simulink library "lib_FDM"  (R2019b)
settings: Solver=VariableStepAuto  StartTime=0.0  StopTime=10.0  RelTol=1e-3
values from neighbouring files (symbols this model uses):
  d = config.d_m    [computeTF.m]
undefined symbols (not defined in the file or in its folder): c_b_WGS, c_flat, c_grav, c_rot, c_rsma, Cd0, Cdcl, Cdcl2, Cl0, Cla, Cld, Cma, Cmd, Cmq, Cnb, Cnd, Cnr, Cra, Crd, Crp, Cy0, Cyb, Cyd, dmdt, Earth, HIL_Data, InitThrust, launchPos, me, mf, mp, Sref, tb, TF, theta0, WGS84
libraries: simulink_extras x14, $bdroot x7, simulink x5, lib_Fin_Deflections x3, aerolibasang x2, sharedtransform x1, aerolibtransform2 x1, aerolibbdyn x1, aerolibatmos2 x1, aerolibutil x1, aerolib6dof2 x1
(part 7 of 8)

== system lib_FDM/FDM/FDM_Sophisticated/stream_flow/calc_stream_flow/velocity_vector_transformation/cross_product ==
  note: Inputs [size]:
      |
      | r1 [3x1]
      | r2 [3x1]
  note: Outputs [size]:
      |
      | r1 x r2  [3x1]
  r1 : Inport
  r2 : Inport  Port=2
  Demux2 : Demux  Outputs=[1;1;1]
  Demux3 : Demux  Outputs=[1;1;1]
  Product{2..7} (6 alike) : Product  SaturateOnIntegerOverflow=on  RndMeth=Zero  InputSameDT=on  OutDataTypeStr=Inherit: Same as first input
  Sum : Sum  Inputs=+-  SaturateOnIntegerOverflow=on  InputSameDT=on  OutDataTypeStr=Inherit: Same as first input
  Sum1 : Sum  Inputs=+-  SaturateOnIntegerOverflow=on  InputSameDT=on  OutDataTypeStr=Inherit: Same as first input
  Sum2 : Sum  Inputs=+-  SaturateOnIntegerOverflow=on  InputSameDT=on  OutDataTypeStr=Inherit: Same as first input
  Vector Concatenate : Concatenate  NumInputs=3  Mode=Multidimensional array
  r1_x_r2 : Outport  PortDimensions=[3,1]  VectorParamsAs1DForOutWhenUnconnected=off
  wires:
  Vector Concatenate/1 -> r1_x_r2/1
  r2/1 -> Demux3/1
  r1/1 -> Demux2/1
  Sum2/1 -> Vector Concatenate/3
  Sum1/1 -> Vector Concatenate/2
  Sum/1 -> Vector Concatenate/1
  Product7/1 -> Sum2/2
  Product6/1 -> Sum2/1
  Product5/1 -> Sum1/2
  Product4/1 -> Sum1/1
  Product3/1 -> Sum/2
  Product2/1 -> Sum/1
  Demux2/1 -> Product5/1, Product6/1
  Demux3/1 -> Product4/2, Product7/2
  Demux2/3 -> Product4/1, Product3/1
  Demux3/2 -> Product3/2, Product6/2
  Demux3/3 -> Product2/2, Product5/2
  Demux2/2 -> Product7/1, Product2/1

== system lib_FDM/FDM/FDM_Sophisticated/tmp/weather/atm_dynamic/trafo_around_z_axis ==
  vec1 : Inport
  gamma : Inport  Port=2
  1_rot_mat : Subsystem  mask(Rotation um 1, 2 oder 3 Achsen){rot_1=Rotation um z-Achse}
      mask prompts: rot_1 "1. Rotation"
      mask help:
      | Dieser Block liefert die Rotationsmatrix T12 für den Fall zurück, dass sich das Ziel-Koordinatensystem (1) durch Drehungen um 1, 2 oder 3 Achsen gegenüber dem Ausgangskoordinatensystem (2) beschreiben lässt (passive Drehung).
      |
      | Die Anzahl der Rotation sowie die Reihenfolge ist frei einstellbar.
      |
      | Die Rotationswinkel haben die Einheit [rad].
      mask TypeOptions rot_1: Rotation um x-Achse | Rotation um y-Achse | Rotation um z-Achse
  Product : Product  Multiplication=Matrix(*)
  Reshape : Reshape  OutputDimensionality=Column vector (2-D)
  vec2 : Outport  VectorParamsAs1DForOutWhenUnconnected=off
  wires:
  Reshape/1 -> Product/2  "vec1"
  vec1/1 -> Reshape/1  "vec1"
  1_rot_mat/1(T12) -> Product/1  "T12"
  gamma/1 -> 1_rot_mat/1(wi1)  "gamma"
  Product/1 -> vec2/1  "vec2"

== system lib_FDM/FDM/FDM_Sophisticated/weight_and_balance/moi/moi_coordinate_transformation/3_rot_mat ==
  wi1 : Inport
  wi2 : Inport  Port=2
  wi3 : Inport  Port=3
  1. Rotation x-Achse : Subsystem
  1. Rotation y-Achse : Subsystem
  1. Rotation z-Achse : Subsystem
  2. Rotation x-Achse : Subsystem
  2. Rotation y-Achse : Subsystem
  2. Rotation z-Achse : Subsystem
  3. Rotation : Product  Inputs=***  Multiplication=Matrix(*)
  3. Rotation x-Achse : Subsystem
  3. Rotation y-Achse : Subsystem
  3. Rotation z-Achse : Subsystem
  Constant : Constant  Value=rot_1
  Constant1 : Constant  Value=rot_2
  Constant2 : Constant  Value=rot_3
  Multiport Switch : MultiPortSwitch
  Multiport Switch1 : MultiPortSwitch
  Multiport Switch2 : MultiPortSwitch
  T12 : Outport  VectorParamsAs1DForOutWhenUnconnected=off
  wires:
  3. Rotation x-Achse/1(3Rot_Matrix_x) -> Multiport Switch2/2
  3. Rotation y-Achse/1(3Rot_Matrix_y) -> Multiport Switch2/3
  2. Rotation z-Achse/1(2Rot_Matrix_z) -> Multiport Switch1/4
  2. Rotation y-Achse/1(2Rot_Matrix_y) -> Multiport Switch1/3
  2. Rotation x-Achse/1(2Rot_Matrix_x) -> Multiport Switch1/2
  3. Rotation/1 -> T12/1  "T12"
  Constant2/1 -> Multiport Switch2/1
  1. Rotation z-Achse/1(1Rot_Matrix_z) -> Multiport Switch/4
  1. Rotation y-Achse/1(1Rot_Matrix_y) -> Multiport Switch/3
  Constant1/1 -> Multiport Switch1/1
  1. Rotation x-Achse/1(1Rot_Matrix_x) -> Multiport Switch/2
  Constant/1 -> Multiport Switch/1
  3. Rotation z-Achse/1(3Rot_Matrix_z) -> Multiport Switch2/4
  wi2/1 -> 2. Rotation x-Achse/1(alpha2), 2. Rotation y-Achse/1(alpha2), 2. Rotation z-Achse/1(alpha2)
  wi1/1 -> 1. Rotation x-Achse/1(alpha1), 1. Rotation y-Achse/1(alpha1), 1. Rotation z-Achse/1(alpha1)
  wi3/1 -> 3. Rotation y-Achse/1(alpha3), 3. Rotation z-Achse/1(alpha3), 3. Rotation x-Achse/1(alpha3)
  Multiport Switch/1 -> 3. Rotation/3
  Multiport Switch1/1 -> 3. Rotation/2
  Multiport Switch2/1 -> 3. Rotation/1

== system lib_FDM/FDM/FDM_Sophisticated/weight_and_balance/moi/steiners_theorem_missile/create_deviation_matrix ==
  pBXB : Inport
  Add : Sum
  Add4 : Sum
  Add5 : Sum
  Demux : Demux  Outputs=3
  Gain : Gain  Gain=-1
  Gain1 : Gain  Gain=-1
  Gain3 : Gain  Gain=-1
  Product{1..6} (6 alike) : Product
  Vector Concatenate1 : Concatenate  NumInputs=3  Mode=Multidimensional array  ConcatenateDimension=2
  Vector Concatenate6 : Concatenate  NumInputs=3
  Vector Concatenate7 : Concatenate  NumInputs=3
  Vector Concatenate8 : Concatenate  NumInputs=3
  T_deviation : Outport  VectorParamsAs1DForOutWhenUnconnected=off
  wires:
  pBXB/1 -> Demux/1
  Vector Concatenate8/1 -> Vector Concatenate1/3
  Product3/1 -> Gain/1
  Product4/1 -> Gain1/1
  Gain1/1 -> Vector Concatenate6/3, Vector Concatenate8/1
  Product2/1 -> Add/2, Add4/1
  Product5/1 -> Add5/2, Add4/2
  Product1/1 -> Add/1, Add5/1
  Add/1 -> Vector Concatenate6/1
  Product6/1 -> Gain3/1
  Add5/1 -> Vector Concatenate7/2
  Demux/2 -> Product6/1, Product1/1, Product1/2, Product3/2  "b"
  Vector Concatenate1/1 -> T_deviation/1
  Gain3/1 -> Vector Concatenate7/3, Vector Concatenate8/2
  Gain/1 -> Vector Concatenate6/2, Vector Concatenate7/1
  Demux/3 -> Product2/2, Product2/1, Product4/2, Product6/2  "c"
  Demux/1 -> Product5/1, Product5/2, Product4/1, Product3/1  "a"
  Vector Concatenate7/1 -> Vector Concatenate1/2
  Vector Concatenate6/1 -> Vector Concatenate1/1
  Add4/1 -> Vector Concatenate8/3

== system lib_FDM/FDM/FDM_Sophisticated/weight_and_balance/moi/steiners_theorem_motor/create_deviation_matrix1 ==
  pBXB : Inport
  Add : Sum
  Add4 : Sum
  Add5 : Sum
  Demux : Demux  Outputs=3
  Gain : Gain  Gain=-1
  Gain1 : Gain  Gain=-1
  Gain3 : Gain  Gain=-1
  Product{1..6} (6 alike) : Product
  Vector Concatenate1 : Concatenate  NumInputs=3  Mode=Multidimensional array  ConcatenateDimension=2
  Vector Concatenate6 : Concatenate  NumInputs=3
  Vector Concatenate7 : Concatenate  NumInputs=3
  Vector Concatenate8 : Concatenate  NumInputs=3
  T_deviation : Outport  VectorParamsAs1DForOutWhenUnconnected=off
  wires:
  Add4/1 -> Vector Concatenate8/3
  Vector Concatenate6/1 -> Vector Concatenate1/1
  Vector Concatenate7/1 -> Vector Concatenate1/2
  Demux/1 -> Product3/1, Product4/1, Product5/2, Product5/1  "a"
  Demux/3 -> Product6/2, Product4/2, Product2/1, Product2/2  "c"
  Gain/1 -> Vector Concatenate7/1, Vector Concatenate6/2
  Gain3/1 -> Vector Concatenate8/2, Vector Concatenate7/3
  Vector Concatenate1/1 -> T_deviation/1
  Demux/2 -> Product3/2, Product1/2, Product1/1, Product6/1  "b"
  Add5/1 -> Vector Concatenate7/2
  Product6/1 -> Gain3/1
  Add/1 -> Vector Concatenate6/1
  Product1/1 -> Add5/1, Add/1
  Product5/1 -> Add4/2, Add5/2
  Product2/1 -> Add4/1, Add/2
  Gain1/1 -> Vector Concatenate8/1, Vector Concatenate6/3
  Product4/1 -> Gain1/1
  Product3/1 -> Gain/1
  Vector Concatenate8/1 -> Vector Concatenate1/3
  pBXB/1 -> Demux/1

== system lib_FDM/FDM/FDM_Student/Aerodynamics/-/Calc Thrust/If Action Subsystem ==
  Action Port : ActionPort
  Constant1 : Constant
  Gain : Gain  Gain=[InitThrust, 0, 0]
  Thrust : Outport  VectorParamsAs1DForOutWhenUnconnected=off
  wires:
  Gain/1 -> Thrust/1
  Constant1/1 -> Gain/1

== system lib_FDM/FDM/FDM_Student/Aerodynamics/-/Calc Thrust/If Action Subsystem1 ==
  Action Port : ActionPort
  Constant1 : Constant
  Gain1 : Gain  Gain=[InitThrust*0, 0, 0]
  Thrust1 : Outport  VectorParamsAs1DForOutWhenUnconnected=off
  wires:
  Constant1/1 -> Gain1/1
  Gain1/1 -> Thrust1/1

== system lib_FDM/FDM/FDM_Student/Aerodynamics/Moment Calc/Calc CL Wind/If Action Subsystem ==
  w_Wind : Inport
  delta R : Inport  Port=2
  AOA : Inport  Port=3
  Vb : Inport  Port=4
  Action Port : ActionPort
  C_L_alpha : Gain  Gain=Cra
  C_L_delta : Gain  Gain=Crd
  C_L_p : Gain  Gain=Crp*0.5*d
  Divide : Product  Inputs=*/
  Selector2 : Selector  InputPortWidth=3  IndexOptions=Index vector (dialog)  Indices=1  OutputSizes=1
  Sum1 : Sum  Inputs=|+++
  To Workspace : ToWorkspace  VariableName=Rolling_moment_wind  SaveFormat=Structure  SampleTime=-1
  CL : Outport  VectorParamsAs1DForOutWhenUnconnected=off
  wires:
  C_L_p/1 -> Divide/1
  Divide/1 -> Sum1/1
  C_L_delta/1 -> Sum1/2
  C_L_alpha/1 -> Sum1/3
  w_Wind/1 -> Selector2/1
  delta R/1 -> C_L_delta/1
  AOA/1 -> C_L_alpha/1
  Vb/1 -> Divide/2
  Selector2/1 -> To Workspace/1, C_L_p/1
  Sum1/1 -> CL/1

== system lib_FDM/FDM/FDM_Student/Aerodynamics/Moment Calc/Calc CL Wind/If Action Subsystem1 ==
  Action Port : ActionPort
  Constant : Constant  Value=0  VectorParams1D=off
  CL : Outport  VectorParamsAs1DForOutWhenUnconnected=off
  wires:
  Constant/1 -> CL/1

== system lib_FDM/FDM/FDM_Student/Aerodynamics/Moment Calc/Calc CM Wind/If Action Subsystem2 ==
  alpha : Inport
  delta p : Inport  Port=2
  w_Wind : Inport  Port=3
  Vb : Inport  Port=4
  Action Port : ActionPort
  C_M_alpha : Gain  Gain=Cma
  C_M_delta : Gain  Gain=Cmd
  C_M_q : Gain  Gain=Cmq*0.5*d
  Divide : Product  Inputs=*/
  Selector1 : Selector  InputPortWidth=3  IndexOptions=Index vector (dialog)  Indices=2  OutputSizes=1
  Sum2 : Sum  Inputs=|+++
  CM : Outport  VectorParamsAs1DForOutWhenUnconnected=off
  wires:
  Sum2/1 -> CM/1
  delta p/1 -> C_M_delta/1
  alpha/1 -> C_M_alpha/1
  C_M_alpha/1 -> Sum2/1
  C_M_q/1 -> Divide/1
  C_M_delta/1 -> Sum2/2
  w_Wind/1 -> Selector1/1
  Selector1/1 -> C_M_q/1
  Divide/1 -> Sum2/3
  Vb/1 -> Divide/2

== system lib_FDM/FDM/FDM_Student/Aerodynamics/Moment Calc/Calc CM Wind/If Action Subsystem3 ==
  Action Port : ActionPort
  Constant : Constant  Value=0  VectorParams1D=off
  CM : Outport  VectorParamsAs1DForOutWhenUnconnected=off
  wires:
  Constant/1 -> CM/1

== system lib_FDM/FDM/FDM_Student/Aerodynamics/Moment Calc/Calc CN Wind/If Action Subsystem2 ==
  beta : Inport
  delta Y : Inport  Port=2
  w_Wind : Inport  Port=3
  Vb : Inport  Port=4
  Action Port : ActionPort
  C_N_beta : Gain  Gain=Cnb
  C_N_delta : Gain  Gain=Cnd
  C_N_r : Gain  Gain=Cnr*0.5*d
  Divide1 : Product  Inputs=*/
  Selector1 : Selector  InputPortWidth=3  IndexOptions=Index vector (dialog)  Indices=3  OutputSizes=1
  Sum : Sum  Inputs=|+++
  CN : Outport  VectorParamsAs1DForOutWhenUnconnected=off
  wires:
  w_Wind/1 -> Selector1/1
  delta Y/1 -> C_N_delta/1
  beta/1 -> C_N_beta/1
  C_N_r/1 -> Divide1/1
  C_N_delta/1 -> Sum/2
  Selector1/1 -> C_N_r/1
  Sum/1 -> CN/1
  C_N_beta/1 -> Sum/1
  Divide1/1 -> Sum/3
  Vb/1 -> Divide1/2

== system lib_FDM/FDM/FDM_Student/Aerodynamics/Moment Calc/Calc CN Wind/If Action Subsystem3 ==
  Action Port : ActionPort
  Constant : Constant  Value=0  VectorParams1D=off
  CN : Outport  VectorParamsAs1DForOutWhenUnconnected=off
  wires:
  Constant/1 -> CN/1

== system lib_FDM/FDM/FDM_Sophisticated/aerodynamics/aerodynamic_via_lookup/calc_aero_for_mom/launch_rail/initial_altitude ==
  Constant : Constant  Value=HIL_Data.FDM.soph.bus2.pBII_0
  Constant2 : Constant  Value=HIL_Data.FDM.soph.bus2.flag_I_flat
  Demux : Demux  Outputs=3
  Gain : Gain  Gain=-1
  Switch1 : Switch  Criteria=u2 > Threshold
  Terminator{,1..3} (4 alike) : Terminator
  trafo_E_to_geodetic : Subsystem  mask(Transformation der ECEF Position in geodätische Größen){}
      mask help: Dieser Block transformiert die Position im ECEF KOS in die geodätische Länge, Breite und Höhe
      mask init:
      | [c_mue, c_rsma, c_flat] = init_transformations_earth;
      mask Help:
      | Name:
      | 
      |     trafo_E_to_geodetic
      | 
      | Beschreibung:
      | 
      |     Dieser Block transformiert die Position im ECEF KOS in die geodätische
      |     Länge, Breite und Höhe.
      | 
      | Inputs   [size]  [data type] [unit]:
      | 
      |     pBEE    [3] [double] [m]
      | 
      | Outputs  [size]  [data type] [unit]:
      | 
      |     long  [1] [double] [rad]
      |     lat   [1] [double] [rad]
      |     alt   [1] [double] [m]
      | 
      | Parameter
      | 
      |    c_rsma
      |    c_flat
  hBE_0 : Outport  VectorParamsAs1DForOutWhenUnconnected=off
  wires:
  Switch1/1 -> hBE_0/1  "hBE_0"
  trafo_E_to_geodetic/1(lon) -> Terminator/1
  Constant/1 -> trafo_E_to_geodetic/1(pBEE), Demux/1
  trafo_E_to_geodetic/2(lat) -> Terminator1/1
  Demux/1 -> Terminator2/1
  Gain/1 -> Switch1/1
  Demux/3 -> Gain/1
  Demux/2 -> Terminator3/1
  trafo_E_to_geodetic/3(alt) -> Switch1/3  "hBE_0"
  Constant2/1 -> Switch1/2

== system lib_FDM/FDM/FDM_Sophisticated/aerodynamics/aerodynamic_via_lookup/calc_aero_for_mom/launch_rail1/initial_altitude ==
  Constant : Constant  Value=HIL_Data.FDM.soph.bus2.pBII_0
  Constant2 : Constant  Value=HIL_Data.FDM.soph.bus2.flag_I_flat
  Demux : Demux  Outputs=3
  Gain : Gain  Gain=-1
  Switch1 : Switch  Criteria=u2 > Threshold
  Terminator{,1..3} (4 alike) : Terminator
  trafo_E_to_geodetic : Subsystem  mask(Transformation der ECEF Position in geodätische Größen){}
      mask help: Dieser Block transformiert die Position im ECEF KOS in die geodätische Länge, Breite und Höhe
      mask init:
      | [c_mue, c_rsma, c_flat] = init_transformations_earth;
      mask Help:
      | Name:
      | 
      |     trafo_E_to_geodetic
      | 
      | Beschreibung:
      | 
      |     Dieser Block transformiert die Position im ECEF KOS in die geodätische
      |     Länge, Breite und Höhe.
      | 
      | Inputs   [size]  [data type] [unit]:
      | 
      |     pBEE    [3] [double] [m]
      | 
      | Outputs  [size]  [data type] [unit]:
      | 
      |     long  [1] [double] [rad]
      |     lat   [1] [double] [rad]
      |     alt   [1] [double] [m]
      | 
      | Parameter
      | 
      |    c_rsma
      |    c_flat
  hBE_0 : Outport  VectorParamsAs1DForOutWhenUnconnected=off
  wires:
  Constant2/1 -> Switch1/2
  trafo_E_to_geodetic/3(alt) -> Switch1/3  "hBE_0"
  Demux/2 -> Terminator3/1
  Demux/3 -> Gain/1
  Gain/1 -> Switch1/1
  Demux/1 -> Terminator2/1
  trafo_E_to_geodetic/2(lat) -> Terminator1/1
  Constant/1 -> Demux/1, trafo_E_to_geodetic/1(pBEE)
  trafo_E_to_geodetic/1(lon) -> Terminator/1
  Switch1/1 -> hBE_0/1  "hBE_0"

== system lib_FDM/FDM/FDM_Sophisticated/environment/WGS84_Gravitation/WGS84_2_ECEF/WGS84 Transformation Parameter /Subsystem ==
  b : Inport
  a : Inport  Port=2
  Add : Sum  Inputs=-+
  Add1 : Sum  Inputs=+-
  Divide : Product  Inputs=*/
  Divide1 : Product  Inputs=**
  Sqrt : Sqrt  SaturateOnIntegerOverflow=on
  a2 : Constant  Value=2
  e : Outport  VectorParamsAs1DForOutWhenUnconnected=off
  wires:
  Add/1 -> Divide/1
  Add1/1 -> Divide1/1
  Divide/1 -> Add1/2, Divide1/2  "f"
  Divide1/1 -> Sqrt/1
  a2/1 -> Add1/1
  b/1 -> Add/1
  a/1 -> Divide/2, Add/2
  Sqrt/1 -> e/1  "e"

== system lib_FDM/FDM/FDM_Sophisticated/gravity/launch_rail/initial_altitude/trafo_E_to_geodetic/Geodetic_altitude ==
  pBEE : Inport
  c_rsma : Inport  Port=2
  c_flat : Inport  Port=3
  lat : Inport  Port=4
  Add : Sum
  Constant : Constant
  Gain : Gain  Gain=2
  Product : Product  Inputs=*/  SaturateOnIntegerOverflow=on  RndMeth=Zero  InputSameDT=on  OutDataTypeStr=Inherit: Same as first input
  Product1 : Product
  Product2 : Product
  Product3 : Product
  Product4 : Product  Inputs=*/  SaturateOnIntegerOverflow=on  RndMeth=Zero  InputSameDT=on  OutDataTypeStr=Inherit: Same as first input
  Product5 : Product  Inputs=3
  Selector : Selector  IndexMode=Zero-based  InputPortWidth=3  IndexOptions=Index vector (dialog)  Indices=0  OutputSizes=1
  Selector1 : Selector  IndexMode=Zero-based  InputPortWidth=3  IndexOptions=Index vector (dialog)  Indices=1  OutputSizes=1
  Sqrt : Sqrt  SaturateOnIntegerOverflow=on
  Sqrt1 : Sqrt  SaturateOnIntegerOverflow=on
  Subtract : Sum  Inputs=+-
  Subtract1 : Sum  Inputs=+-
  Sum : Sum  Inputs=+-  SaturateOnIntegerOverflow=on  InputSameDT=on  OutDataTypeStr=Inherit: Same as first input
  Trigonometric Function : Trigonometry
  cos(latGD) : Trigonometry  Operator=cos
  alt : Outport  VectorParamsAs1DForOutWhenUnconnected=off
  wires:
  lat/1 -> Trigonometric Function/1, cos(latGD)/1
  Sqrt/1 -> Product/1
  cos(latGD)/1 -> Product/2
  c_rsma/1 -> Product4/1
  Subtract/1 -> Product5/3
  Product/1 -> Sum/1
  Sum/1 -> alt/1  "alt"
  Selector/1 -> Product1/2, Product1/1
  Selector1/1 -> Product2/2, Product2/1
  Product1/1 -> Add/1
  Product2/1 -> Add/2
  Add/1 -> Sqrt/1
  pBEE/1 -> Selector1/1, Selector/1
  Product3/1 -> Subtract/2
  Gain/1 -> Subtract/1
  c_flat/1 -> Product3/1, Product3/2, Gain/1
  Sqrt1/1 -> Product4/2
  Subtract1/1 -> Sqrt1/1
  Constant/1 -> Subtract1/1
  Product5/1 -> Subtract1/2
  Trigonometric Function/1 -> Product5/2, Product5/1
  Product4/1 -> Sum/2

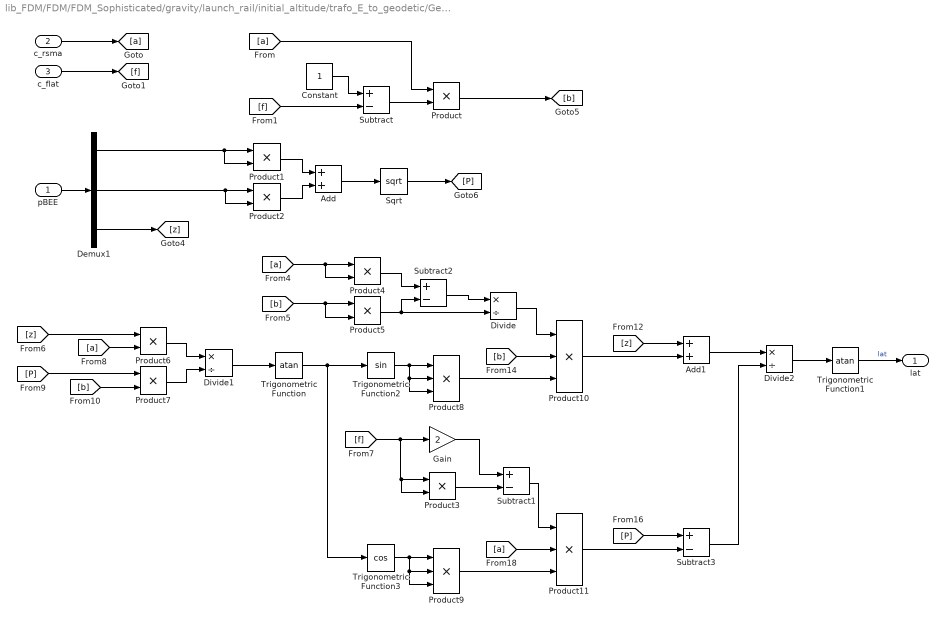
== system lib_FDM/FDM/FDM_Sophisticated/gravity/launch_rail/initial_altitude/trafo_E_to_geodetic/Geodetic_latitude ==
  pBEE : Inport
  c_rsma : Inport  Port=2
  c_flat : Inport  Port=3
  Add : Sum
  Add1 : Sum
  Constant : Constant
  Demux1 : Demux  Outputs=[1;1;1]
  Divide : Product  Inputs=*/
  Divide1 : Product  Inputs=*/
  Divide2 : Product  Inputs=*/
  Gain : Gain  Gain=2
  Product{,1..7} (8 alike) : Product
  Product{8..11} (4 alike) : Product  Inputs=3
  Sqrt : Sqrt  SaturateOnIntegerOverflow=on
  Subtract{,1..3} (4 alike) : Sum  Inputs=+-
  Trigonometric Function : Trigonometry  Operator=atan
  Trigonometric Function1 : Trigonometry  Operator=atan
  Trigonometric Function2 : Trigonometry
  Trigonometric Function3 : Trigonometry  Operator=cos
  lat : Outport  VectorParamsAs1DForOutWhenUnconnected=off
  wires:
  c_flat/1 -> [f]
  c_rsma/1 -> [a]
  pBEE/1 -> Demux1/1
  Demux1/3 -> [z]
  [a] -> Product/1
  [f] -> Subtract/2
  Demux1/1 -> Product1/2, Product1/1
  Demux1/2 -> Product2/2, Product2/1
  [a] -> Product4/2, Product4/1
  [b] -> Product5/2, Product5/1
  [f] -> Product3/2, Product3/1, Gain/1
  [z] -> Product6/1
  [a] -> Product6/2
  Trigonometric Function/1 -> Trigonometric Function3/1, Trigonometric Function2/1
  [P] -> Product7/1
  [b] -> Product7/2
  [z] -> Add1/1
  [b] -> Product10/2
  [P] -> Subtract3/1
  Subtract1/1 -> Product11/1
  [a] -> Product11/2
  Trigonometric Function1/1 -> lat/1  "lat"
  Constant/1 -> Subtract/1
  Subtract/1 -> Product/2
  Product/1 -> [b]
  Product1/1 -> Add/1
  Product2/1 -> Add/2
  Add/1 -> Sqrt/1
  Sqrt/1 -> [P]
  Product3/1 -> Subtract1/2
  Gain/1 -> Subtract1/1
  Product4/1 -> Subtract2/1
  Product5/1 -> Subtract2/2, Divide/2
  Subtract2/1 -> Divide/1
  Product6/1 -> Divide1/1
  Product7/1 -> Divide1/2
  Divide1/1 -> Trigonometric Function/1
  Divide2/1 -> Trigonometric Function1/1
  Trigonometric Function2/1 -> Product8/2, Product8/3, Product8/1
  Trigonometric Function3/1 -> Product9/2, Product9/3, Product9/1
  Product8/1 -> Product10/3
  Product10/1 -> Add1/2
  Add1/1 -> Divide2/1
  Subtract3/1 -> Divide2/2
  Product11/1 -> Subtract3/2
  Product9/1 -> Product11/3
  Divide/1 -> Product10/1

== system lib_FDM/FDM/FDM_Sophisticated/motion_kinematics/calc_motion_kinematics/calc_transformation_matrix/q31_from_q32_mul_q1/normalize_quaternion ==
  note: Inputs [size]:
      |
      | q [4]
  note: Outputs [size]:
      |
      | q_norm [4]
  q : Inport
  Add : Sum  Inputs=++++
  Demux : Demux  Outputs=[1;1;1;1]
  Math Function : Math  Operator=sqrt  SaturateOnIntegerOverflow=on
  Product : Product  Inputs=*/  SaturateOnIntegerOverflow=on  RndMeth=Zero  InputSameDT=on  OutDataTypeStr=Inherit: Same as first input
  Product{1..4} (4 alike) : Product  RndMeth=Zero
  q_normalized : Outport  VectorParamsAs1DForOutWhenUnconnected=off
  wires:
  Product/1 -> q_normalized/1
  q/1 -> Product/1, Demux/1
  Demux/1 -> Product1/1, Product1/2
  Demux/2 -> Product2/1, Product2/2
  Demux/3 -> Product3/1, Product3/2
  Demux/4 -> Product4/1, Product4/2
  Product4/1 -> Add/4
  Product3/1 -> Add/3
  Product2/1 -> Add/2
  Product1/1 -> Add/1
  Add/1 -> Math Function/1
  Math Function/1 -> Product/2

== system lib_FDM/FDM/FDM_Sophisticated/motion_kinematics/calc_motion_kinematics/calc_transformation_matrix/q31_from_q32_mul_q2/normalize_quaternion ==
  note: Inputs [size]:
      |
      | q [4]
  note: Outputs [size]:
      |
      | q_norm [4]
  q : Inport
  Add : Sum  Inputs=++++
  Demux : Demux  Outputs=[1;1;1;1]
  Math Function : Math  Operator=sqrt  SaturateOnIntegerOverflow=on
  Product : Product  Inputs=*/  SaturateOnIntegerOverflow=on  RndMeth=Zero  InputSameDT=on  OutDataTypeStr=Inherit: Same as first input
  Product{1..4} (4 alike) : Product  RndMeth=Zero
  q_normalized : Outport  VectorParamsAs1DForOutWhenUnconnected=off
  wires:
  Product/1 -> q_normalized/1
  q/1 -> Product/1, Demux/1
  Demux/1 -> Product1/1, Product1/2
  Demux/2 -> Product2/1, Product2/2
  Demux/3 -> Product3/1, Product3/2
  Demux/4 -> Product4/1, Product4/2
  Product4/1 -> Add/4
  Product3/1 -> Add/3
  Product2/1 -> Add/2
  Product1/1 -> Add/1
  Add/1 -> Math Function/1
  Math Function/1 -> Product/2

== system lib_FDM/FDM/FDM_Sophisticated/motion_kinematics/calc_motion_kinematics/calc_transformation_matrix/q31_from_q32_mul_q21/normalize_quaternion ==
  note: Inputs [size]:
      |
      | q [4]
  note: Outputs [size]:
      |
      | q_norm [4]
  q : Inport
  Add : Sum  Inputs=++++
  Demux : Demux  Outputs=[1;1;1;1]
  Math Function : Math  Operator=sqrt  SaturateOnIntegerOverflow=on
  Product : Product  Inputs=*/  SaturateOnIntegerOverflow=on  RndMeth=Zero  InputSameDT=on  OutDataTypeStr=Inherit: Same as first input
  Product{1..4} (4 alike) : Product  RndMeth=Zero
  q_normalized : Outport  VectorParamsAs1DForOutWhenUnconnected=off
  wires:
  Product/1 -> q_normalized/1
  q/1 -> Product/1, Demux/1
  Demux/1 -> Product1/1, Product1/2
  Demux/2 -> Product2/1, Product2/2
  Demux/3 -> Product3/1, Product3/2
  Demux/4 -> Product4/1, Product4/2
  Product4/1 -> Add/4
  Product3/1 -> Add/3
  Product2/1 -> Add/2
  Product1/1 -> Add/1
  Add/1 -> Math Function/1
  Math Function/1 -> Product/2

== system lib_FDM/FDM/FDM_Sophisticated/motion_kinematics/calc_motion_kinematics/earth_rotation/quaternion_integration/Subsystem1 ==
  wEIE : Inport
  qIE : Inport  Port=2
  Add : Sum  Inputs=4
  Constant8 : Constant  Value=0
  Demux : Demux
  Demux1 : Demux  Outputs=3
  Gain : Gain  Gain=0.5
  Product{1..4} (4 alike) : Product
  Product5 : Product  Multiplication=Matrix(*)
  Q_1 : Constant  Value=[0 0 0 1; 0 0 1 0; 0 -1 0 0; -1 0 0 0]
  Q_2 : Constant  Value=[0 0 -1 0; 0 0 0 1; 1 0 0 0; 0 -1 0 0]
  Q_3 : Constant  Value=[0 1 0 0; -1 0 0 0; 0 0 0 1; 0 0 -1 0]
  Q_4 : Constant  Value=[1 0 0 0; 0 1 0 0; 0 0 1 0; 0 0 0 1]
  Vector Concatenate : Concatenate  NumInputs=4
  conjugate_quaternion1 : Subsystem
      mask help: conjugate a quaternion
      mask Help:
      | Name:
      | 
      |     conjugate_quaternion
      | 
      | Description:
      | 
      |     computes the conjugate quaternion
      | 
      | Inputs  [size] [data type] [unit]:
      | 
      |     quaternion q_2_1  [4] [double] [-]
      | 
      | Outputs  [size] [data type] [unit]:
      | 
      |     conjugated quaternion q_1_2  [4] [double] [-]
      mask Display: disp (' conj(q)')
  conjugate_quaternion2 : Subsystem
      mask help: conjugate a quaternion
      mask Help:
      | Name:
      | 
      |     conjugate_quaternion
      | 
      | Description:
      | 
      |     computes the conjugate quaternion
      | 
      | Inputs  [size] [data type] [unit]:
      | 
      |     quaternion q_2_1  [4] [double] [-]
      | 
      | Outputs  [size] [data type] [unit]:
      | 
      |     conjugated quaternion q_1_2  [4] [double] [-]
      mask Display: disp (' conj(q)')
  d_qIE : Outport  VectorParamsAs1DForOutWhenUnconnected=off
  wires:
  conjugate_quaternion2/1(q_conj) -> d_qIE/1  "d_qIE"
  wEIE/1 -> Demux1/1
  Demux/2 -> Product2/2  "w2"
  conjugate_quaternion1/1(q_conj) -> Product5/2  "qEI"
  Demux1/2 -> Vector Concatenate/2
  Demux/3 -> Product3/2  "w3"
  Q_4/1 -> Product4/1
  Product1/1 -> Add/1
  Gain/1 -> conjugate_quaternion2/1(q)  "d_qEI"
  Product5/1 -> Gain/1
  Q_2/1 -> Product2/1
  Vector Concatenate/1 -> Demux/1
  Demux/1 -> Product1/2  "w1"
  Demux1/1 -> Vector Concatenate/1
  Constant8/1 -> Vector Concatenate/4
  Q_1/1 -> Product1/1
  Q_3/1 -> Product3/1
  Product3/1 -> Add/3
  Product4/1 -> Add/4
  Demux/4 -> Product4/2  "w4"
  Add/1 -> Product5/1
  Product2/1 -> Add/2
  Demux1/3 -> Vector Concatenate/3
  qIE/1 -> conjugate_quaternion1/1(q)

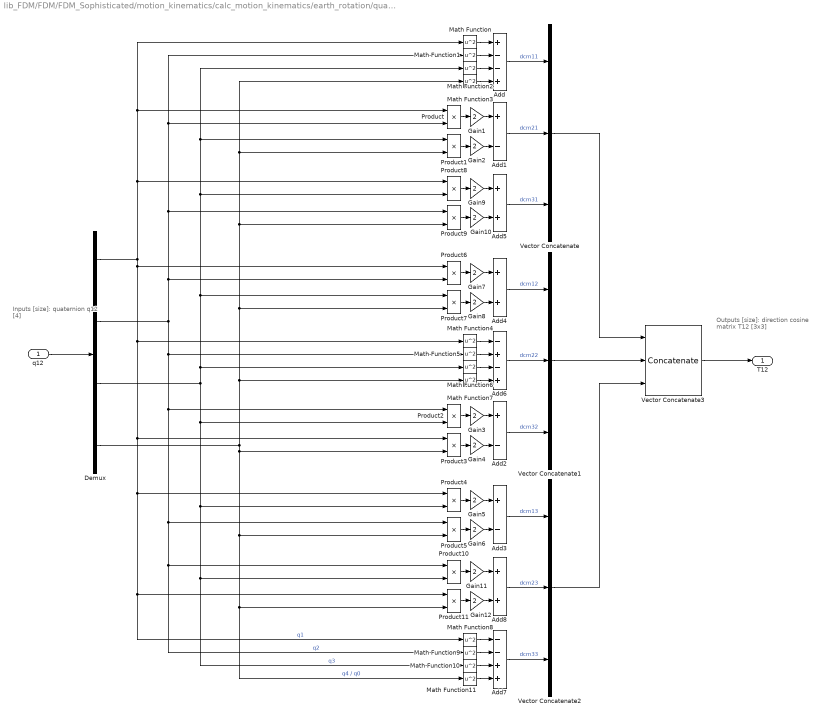
== system lib_FDM/FDM/FDM_Sophisticated/motion_kinematics/calc_motion_kinematics/earth_rotation/quaternion_integration/T12_from_q12 ==
  note: Outputs [size]:
      |
      | direction cosine matrix T12 [3x3]
  note: Inputs [size]:
      |
      | quaternion q12 [4]
  q12 : Inport  PortDimensions=4
  Add : Sum  Inputs=+--+
  Add1 : Sum  Inputs=+-
  Add2 : Sum  Inputs=+-
  Add3 : Sum  Inputs=+-
  Add4 : Sum
  Add5 : Sum
  Add6 : Sum  Inputs=-+-+
  Add7 : Sum  Inputs=--++
  Add8 : Sum
  Demux : Demux
  Gain{1..12} (12 alike) : Gain  Gain=2
  Math Function{,1..11} (12 alike) : Math  Operator=square  SaturateOnIntegerOverflow=on
  Product{,1..11} (12 alike) : Product
  Vector Concatenate : Concatenate  NumInputs=3
  Vector Concatenate1 : Concatenate  NumInputs=3
  Vector Concatenate2 : Concatenate  NumInputs=3
  Vector Concatenate3 : Concatenate  NumInputs=3  Mode=Multidimensional array  ConcatenateDimension=2
  T12 : Outport  PortDimensions=[3 3]  VectorParamsAs1DForOutWhenUnconnected=off
  wires:
  q12/1 -> Demux/1
  Demux/1 -> Product8/1, Product/1, Math Function/1, Product3/1, Product4/1, Product11/1, Math Function8/1, Math Function4/1, Product6/1  "q1"
  Demux/2 -> Product2/1, Product5/1, Product10/1, Math Function9/1, Math Function5/1, Product6/2, Product9/1, Product/2, Math Function1/1  "q2"
  Demux/3 -> Product2/2, Product4/2, Math Function10/1, Product10/2, Math Function6/1, Product7/1, Product8/2, Product1/1, Math Function2/1  "q3"
  Demux/4 -> Math Function7/1, Product7/2, Product9/2, Product1/2, Math Function3/1, Product5/2, Math Function11/1, Product11/2, Product3/2  "q4 / q0"
  Vector Concatenate3/1 -> T12/1
  Vector Concatenate/1 -> Vector Concatenate3/1
  Vector Concatenate2/1 -> Vector Concatenate3/3
  Vector Concatenate1/1 -> Vector Concatenate3/2
  Add/1 -> Vector Concatenate/1  "dcm11"
  Add1/1 -> Vector Concatenate/2  "dcm21"
  Add5/1 -> Vector Concatenate/3  "dcm31"
  Add4/1 -> Vector Concatenate1/1  "dcm12"
  Add6/1 -> Vector Concatenate1/2  "dcm22"
  Add2/1 -> Vector Concatenate1/3  "dcm32"
  Add3/1 -> Vector Concatenate2/1  "dcm13"
  Add8/1 -> Vector Concatenate2/2  "dcm23"
  Add7/1 -> Vector Concatenate2/3  "dcm33"
  Math Function/1 -> Add/1
  Math Function1/1 -> Add/2
  Math Function2/1 -> Add/3
  Math Function3/1 -> Add/4
  Product/1 -> Gain1/1
  Product1/1 -> Gain2/1
  Gain1/1 -> Add1/1
  Gain2/1 -> Add1/2
  Gain4/1 -> Add2/2
  Gain3/1 -> Add2/1
  Product3/1 -> Gain4/1
  Product2/1 -> Gain3/1
  Gain6/1 -> Add3/2
  Gain5/1 -> Add3/1
  Product5/1 -> Gain6/1
  Product4/1 -> Gain5/1
  Gain8/1 -> Add4/2
  Gain7/1 -> Add4/1
  Product7/1 -> Gain8/1
  Product6/1 -> Gain7/1
  Gain10/1 -> Add5/2
  Gain9/1 -> Add5/1
  Product9/1 -> Gain10/1
  Product8/1 -> Gain9/1
  Math Function6/1 -> Add6/3
  Math Function7/1 -> Add6/4
  Math Function5/1 -> Add6/2
  Math Function4/1 -> Add6/1
  Math Function10/1 -> Add7/3
  Math Function11/1 -> Add7/4
  Math Function9/1 -> Add7/2
  Math Function8/1 -> Add7/1
  Gain12/1 -> Add8/2
  Gain11/1 -> Add8/1
  Product11/1 -> Gain12/1
  Product10/1 -> Gain11/1

== system lib_FDM/FDM/FDM_Sophisticated/motion_kinematics/calc_motion_kinematics/earth_rotation/quaternion_integration1/Subsystem1 ==
  wGEG : Inport
  qEG : Inport  Port=2
  Add : Sum  Inputs=4
  Constant8 : Constant  Value=0
  Demux : Demux
  Demux1 : Demux  Outputs=3
  Gain : Gain  Gain=0.5
  Product{1..4} (4 alike) : Product
  Product5 : Product  Multiplication=Matrix(*)
  Q_1 : Constant  Value=[0 0 0 1; 0 0 1 0; 0 -1 0 0; -1 0 0 0]
  Q_2 : Constant  Value=[0 0 -1 0; 0 0 0 1; 1 0 0 0; 0 -1 0 0]
  Q_3 : Constant  Value=[0 1 0 0; -1 0 0 0; 0 0 0 1; 0 0 -1 0]
  Q_4 : Constant  Value=[1 0 0 0; 0 1 0 0; 0 0 1 0; 0 0 0 1]
  Vector Concatenate : Concatenate  NumInputs=4
  conjugate_quaternion1 : Subsystem
      mask help: conjugate a quaternion
      mask Help:
      | Name:
      | 
      |     conjugate_quaternion
      | 
      | Description:
      | 
      |     computes the conjugate quaternion
      | 
      | Inputs  [size] [data type] [unit]:
      | 
      |     quaternion q_2_1  [4] [double] [-]
      | 
      | Outputs  [size] [data type] [unit]:
      | 
      |     conjugated quaternion q_1_2  [4] [double] [-]
      mask Display: disp (' conj(q)')
  conjugate_quaternion2 : Subsystem
      mask help: conjugate a quaternion
      mask Help:
      | Name:
      | 
      |     conjugate_quaternion
      | 
      | Description:
      | 
      |     computes the conjugate quaternion
      | 
      | Inputs  [size] [data type] [unit]:
      | 
      |     quaternion q_2_1  [4] [double] [-]
      | 
      | Outputs  [size] [data type] [unit]:
      | 
      |     conjugated quaternion q_1_2  [4] [double] [-]
      mask Display: disp (' conj(q)')
  d_qEG : Outport  VectorParamsAs1DForOutWhenUnconnected=off
  wires:
  qEG/1 -> conjugate_quaternion1/1(q)
  Demux1/3 -> Vector Concatenate/3
  Product2/1 -> Add/2
  Add/1 -> Product5/1
  Demux/4 -> Product4/2  "w4"
  Product4/1 -> Add/4
  Product3/1 -> Add/3
  Q_3/1 -> Product3/1
  Q_1/1 -> Product1/1
  Constant8/1 -> Vector Concatenate/4
  Demux1/1 -> Vector Concatenate/1
  Demux/1 -> Product1/2  "w1"
  Vector Concatenate/1 -> Demux/1
  Q_2/1 -> Product2/1
  Product5/1 -> Gain/1
  Gain/1 -> conjugate_quaternion2/1(q)  "d_qGE"
  Product1/1 -> Add/1
  Q_4/1 -> Product4/1
  Demux/3 -> Product3/2  "w3"
  Demux1/2 -> Vector Concatenate/2
  conjugate_quaternion1/1(q_conj) -> Product5/2  "qGE"
  Demux/2 -> Product2/2  "w2"
  wGEG/1 -> Demux1/1
  conjugate_quaternion2/1(q_conj) -> d_qEG/1  "d_qEG"

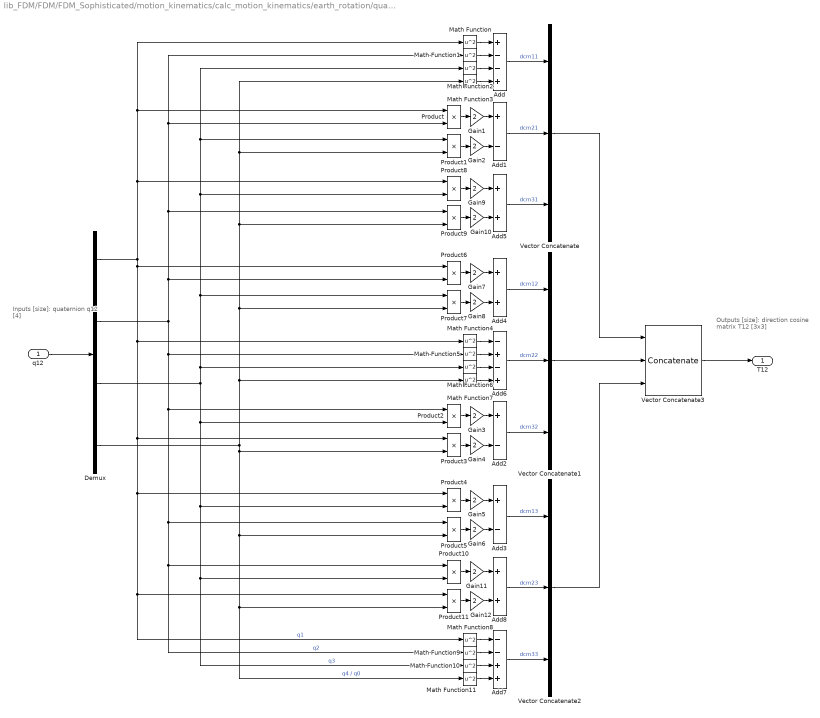
== system lib_FDM/FDM/FDM_Sophisticated/motion_kinematics/calc_motion_kinematics/earth_rotation/quaternion_integration1/T12_from_q12 ==
  note: Outputs [size]:
      |
      | direction cosine matrix T12 [3x3]
  note: Inputs [size]:
      |
      | quaternion q12 [4]
  q12 : Inport  PortDimensions=4
  Add : Sum  Inputs=+--+
  Add1 : Sum  Inputs=+-
  Add2 : Sum  Inputs=+-
  Add3 : Sum  Inputs=+-
  Add4 : Sum
  Add5 : Sum
  Add6 : Sum  Inputs=-+-+
  Add7 : Sum  Inputs=--++
  Add8 : Sum
  Demux : Demux
  Gain{1..12} (12 alike) : Gain  Gain=2
  Math Function{,1..11} (12 alike) : Math  Operator=square  SaturateOnIntegerOverflow=on
  Product{,1..11} (12 alike) : Product
  Vector Concatenate : Concatenate  NumInputs=3
  Vector Concatenate1 : Concatenate  NumInputs=3
  Vector Concatenate2 : Concatenate  NumInputs=3
  Vector Concatenate3 : Concatenate  NumInputs=3  Mode=Multidimensional array  ConcatenateDimension=2
  T12 : Outport  PortDimensions=[3 3]  VectorParamsAs1DForOutWhenUnconnected=off
  wires:
  q12/1 -> Demux/1
  Demux/1 -> Product8/1, Product/1, Math Function/1, Product3/1, Product4/1, Product11/1, Math Function8/1, Math Function4/1, Product6/1  "q1"
  Demux/2 -> Product2/1, Product5/1, Product10/1, Math Function9/1, Math Function5/1, Product6/2, Product9/1, Product/2, Math Function1/1  "q2"
  Demux/3 -> Product2/2, Product4/2, Math Function10/1, Product10/2, Math Function6/1, Product7/1, Product8/2, Product1/1, Math Function2/1  "q3"
  Demux/4 -> Math Function7/1, Product7/2, Product9/2, Product1/2, Math Function3/1, Product5/2, Math Function11/1, Product11/2, Product3/2  "q4 / q0"
  Vector Concatenate3/1 -> T12/1
  Vector Concatenate/1 -> Vector Concatenate3/1
  Vector Concatenate2/1 -> Vector Concatenate3/3
  Vector Concatenate1/1 -> Vector Concatenate3/2
  Add/1 -> Vector Concatenate/1  "dcm11"
  Add1/1 -> Vector Concatenate/2  "dcm21"
  Add5/1 -> Vector Concatenate/3  "dcm31"
  Add4/1 -> Vector Concatenate1/1  "dcm12"
  Add6/1 -> Vector Concatenate1/2  "dcm22"
  Add2/1 -> Vector Concatenate1/3  "dcm32"
  Add3/1 -> Vector Concatenate2/1  "dcm13"
  Add8/1 -> Vector Concatenate2/2  "dcm23"
  Add7/1 -> Vector Concatenate2/3  "dcm33"
  Math Function/1 -> Add/1
  Math Function1/1 -> Add/2
  Math Function2/1 -> Add/3
  Math Function3/1 -> Add/4
  Product/1 -> Gain1/1
  Product1/1 -> Gain2/1
  Gain1/1 -> Add1/1
  Gain2/1 -> Add1/2
  Gain4/1 -> Add2/2
  Gain3/1 -> Add2/1
  Product3/1 -> Gain4/1
  Product2/1 -> Gain3/1
  Gain6/1 -> Add3/2
  Gain5/1 -> Add3/1
  Product5/1 -> Gain6/1
  Product4/1 -> Gain5/1
  Gain8/1 -> Add4/2
  Gain7/1 -> Add4/1
  Product7/1 -> Gain8/1
  Product6/1 -> Gain7/1
  Gain10/1 -> Add5/2
  Gain9/1 -> Add5/1
  Product9/1 -> Gain10/1
  Product8/1 -> Gain9/1
  Math Function6/1 -> Add6/3
  Math Function7/1 -> Add6/4
  Math Function5/1 -> Add6/2
  Math Function4/1 -> Add6/1
  Math Function10/1 -> Add7/3
  Math Function11/1 -> Add7/4
  Math Function9/1 -> Add7/2
  Math Function8/1 -> Add7/1
  Gain12/1 -> Add8/2
  Gain11/1 -> Add8/1
  Product11/1 -> Gain12/1
  Product10/1 -> Gain11/1

== system lib_FDM/FDM/FDM_Sophisticated/rb_eom/calc_bus_flight_dyn_bus_entries/Subsystem2/trafo_E_to_geodetic/Geodetic_altitude ==
  pBEE : Inport
  c_rsma : Inport  Port=2
  c_flat : Inport  Port=3
  lat : Inport  Port=4
  Add : Sum
  Constant : Constant
  Gain : Gain  Gain=2
  Product : Product  Inputs=*/  SaturateOnIntegerOverflow=on  RndMeth=Zero  InputSameDT=on  OutDataTypeStr=Inherit: Same as first input
  Product1 : Product
  Product2 : Product
  Product3 : Product
  Product4 : Product  Inputs=*/  SaturateOnIntegerOverflow=on  RndMeth=Zero  InputSameDT=on  OutDataTypeStr=Inherit: Same as first input
  Product5 : Product  Inputs=3
  Selector : Selector  IndexMode=Zero-based  InputPortWidth=3  IndexOptions=Index vector (dialog)  Indices=0  OutputSizes=1
  Selector1 : Selector  IndexMode=Zero-based  InputPortWidth=3  IndexOptions=Index vector (dialog)  Indices=1  OutputSizes=1
  Sqrt : Sqrt  SaturateOnIntegerOverflow=on
  Sqrt1 : Sqrt  SaturateOnIntegerOverflow=on
  Subtract : Sum  Inputs=+-
  Subtract1 : Sum  Inputs=+-
  Sum : Sum  Inputs=+-  SaturateOnIntegerOverflow=on  InputSameDT=on  OutDataTypeStr=Inherit: Same as first input
  Trigonometric Function : Trigonometry
  cos(latGD) : Trigonometry  Operator=cos
  alt : Outport  VectorParamsAs1DForOutWhenUnconnected=off
  wires:
  lat/1 -> Trigonometric Function/1, cos(latGD)/1
  Sqrt/1 -> Product/1
  cos(latGD)/1 -> Product/2
  c_rsma/1 -> Product4/1
  Subtract/1 -> Product5/3
  Product/1 -> Sum/1
  Sum/1 -> alt/1  "alt"
  Selector/1 -> Product1/2, Product1/1
  Selector1/1 -> Product2/2, Product2/1
  Product1/1 -> Add/1
  Product2/1 -> Add/2
  Add/1 -> Sqrt/1
  pBEE/1 -> Selector1/1, Selector/1
  Product3/1 -> Subtract/2
  Gain/1 -> Subtract/1
  c_flat/1 -> Product3/1, Product3/2, Gain/1
  Sqrt1/1 -> Product4/2
  Subtract1/1 -> Sqrt1/1
  Constant/1 -> Subtract1/1
  Product5/1 -> Subtract1/2
  Trigonometric Function/1 -> Product5/2, Product5/1
  Product4/1 -> Sum/2

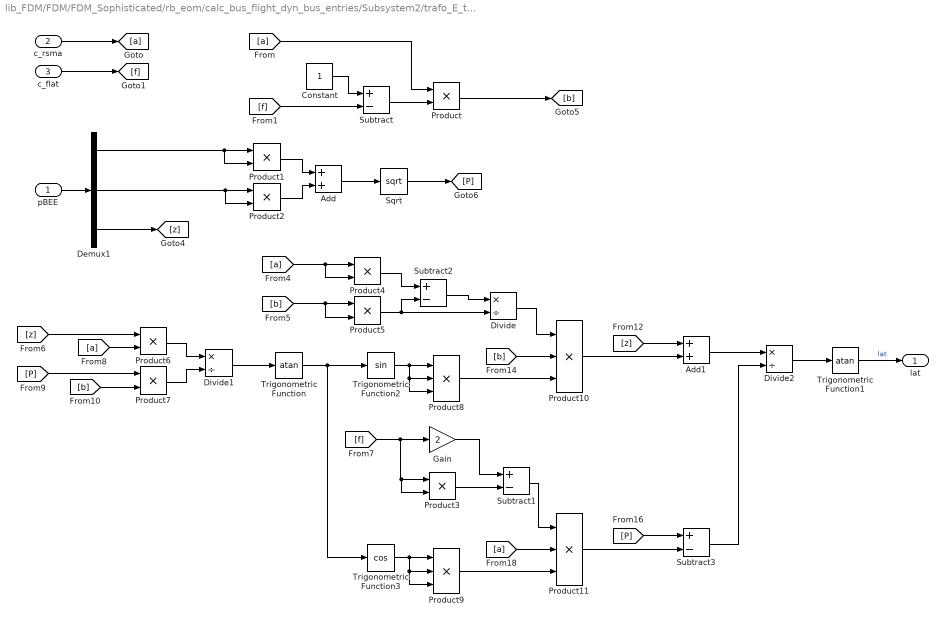
== system lib_FDM/FDM/FDM_Sophisticated/rb_eom/calc_bus_flight_dyn_bus_entries/Subsystem2/trafo_E_to_geodetic/Geodetic_latitude ==
  pBEE : Inport
  c_rsma : Inport  Port=2
  c_flat : Inport  Port=3
  Add : Sum
  Add1 : Sum
  Constant : Constant
  Demux1 : Demux  Outputs=[1;1;1]
  Divide : Product  Inputs=*/
  Divide1 : Product  Inputs=*/
  Divide2 : Product  Inputs=*/
  Gain : Gain  Gain=2
  Product{,1..7} (8 alike) : Product
  Product{8..11} (4 alike) : Product  Inputs=3
  Sqrt : Sqrt  SaturateOnIntegerOverflow=on
  Subtract{,1..3} (4 alike) : Sum  Inputs=+-
  Trigonometric Function : Trigonometry  Operator=atan
  Trigonometric Function1 : Trigonometry  Operator=atan
  Trigonometric Function2 : Trigonometry
  Trigonometric Function3 : Trigonometry  Operator=cos
  lat : Outport  VectorParamsAs1DForOutWhenUnconnected=off
  wires:
  c_flat/1 -> [f]
  c_rsma/1 -> [a]
  pBEE/1 -> Demux1/1
  Demux1/3 -> [z]
  [a] -> Product/1
  [f] -> Subtract/2
  Demux1/1 -> Product1/2, Product1/1
  Demux1/2 -> Product2/2, Product2/1
  [a] -> Product4/2, Product4/1
  [b] -> Product5/2, Product5/1
  [f] -> Product3/2, Product3/1, Gain/1
  [z] -> Product6/1
  [a] -> Product6/2
  Trigonometric Function/1 -> Trigonometric Function3/1, Trigonometric Function2/1
  [P] -> Product7/1
  [b] -> Product7/2
  [z] -> Add1/1
  [b] -> Product10/2
  [P] -> Subtract3/1
  Subtract1/1 -> Product11/1
  [a] -> Product11/2
  Trigonometric Function1/1 -> lat/1  "lat"
  Constant/1 -> Subtract/1
  Subtract/1 -> Product/2
  Product/1 -> [b]
  Product1/1 -> Add/1
  Product2/1 -> Add/2
  Add/1 -> Sqrt/1
  Sqrt/1 -> [P]
  Product3/1 -> Subtract1/2
  Gain/1 -> Subtract1/1
  Product4/1 -> Subtract2/1
  Product5/1 -> Subtract2/2, Divide/2
  Subtract2/1 -> Divide/1
  Product6/1 -> Divide1/1
  Product7/1 -> Divide1/2
  Divide1/1 -> Trigonometric Function/1
  Divide2/1 -> Trigonometric Function1/1
  Trigonometric Function2/1 -> Product8/2, Product8/3, Product8/1
  Trigonometric Function3/1 -> Product9/2, Product9/3, Product9/1
  Product8/1 -> Product10/3
  Product10/1 -> Add1/2
  Add1/1 -> Divide2/1
  Subtract3/1 -> Divide2/2
  Product11/1 -> Subtract3/2
  Product9/1 -> Product11/3
  Divide/1 -> Product10/1

== system lib_FDM/FDM/FDM_Sophisticated/rb_eom/eom_6dof/Rigid_Body_EOM_6_DOF/Integration/normalize_quaternion ==
  note: Inputs [size]:
      |
      | q [4]
  note: Outputs [size]:
      |
      | q_norm [4]
  q : Inport
  Add : Sum  Inputs=++++
  Demux : Demux  Outputs=[1;1;1;1]
  Math Function : Math  Operator=sqrt  SaturateOnIntegerOverflow=on
  Product : Product  Inputs=*/  SaturateOnIntegerOverflow=on  RndMeth=Zero  InputSameDT=on  OutDataTypeStr=Inherit: Same as first input
  Product{1..4} (4 alike) : Product  RndMeth=Zero
  q_normalized : Outport  VectorParamsAs1DForOutWhenUnconnected=off
  wires:
  Product/1 -> q_normalized/1
  q/1 -> Product/1, Demux/1
  Demux/1 -> Product1/1, Product1/2
  Demux/2 -> Product2/1, Product2/2
  Demux/3 -> Product3/1, Product3/2
  Demux/4 -> Product4/1, Product4/2
  Product4/1 -> Add/4
  Product3/1 -> Add/3
  Product2/1 -> Add/2
  Product1/1 -> Add/1
  Add/1 -> Math Function/1
  Math Function/1 -> Product/2

== system lib_FDM/FDM/FDM_Sophisticated/rb_eom/eom_6dof/Rigid_Body_EOM_6_DOF/rb_eom_6dof/calc_d_qIB ==
  note: Body-Drehraten
      | d_qBI(1) =1/2 { q4wx  - q3wy + q2wz }
      | d_qBI(2) =1/2 { q3wx + q4wy  - q1wz }
      | d_qBI(3) =1/2 {-q2wx + q1wy + q4wz }
      | d_qBI(4) =1/2 {-q1wx  - q2wy  - q3wz }
      |
      | Entspricht Zipfel (s. 372, Gl 10.11)
      | Entspricht "Representing Attitude: Euler angles, Unit Quaternions, and Rotation Vectors",
      | 	J. Diebel, Stanford University, S. 16, Gl 157 oder (159 & 151)
      |
      | d_qBI = 1/2 * [wBIB (1, 2, 3), 0] * qBI
  qIB : Inport
  wBIB : Inport  Port=2
  Add : Sum  Inputs=++++
  Constant : Constant  Value=0
  Demux : Demux  Outputs=3
  Demux1 : Demux
  Gain : Gain  Gain=0.5
  Product{2..5} (4 alike) : Product
  Product6 : Product  Multiplication=Matrix(*)
  Q_1 : Constant  Value=[0 0 0 1; 0 0 1 0; 0 -1 0 0; -1 0 0 0]
  Q_2 : Constant  Value=[0 0 -1 0; 0 0 0 1; 1 0 0 0; 0 -1 0 0]
  Q_3 : Constant  Value=[0 1 0 0; -1 0 0 0; 0 0 0 1; 0 0 -1 0]
  Q_4 : Constant  Value=[1 0 0 0; 0 1 0 0; 0 0 1 0; 0 0 0 1]
  Vector Concatenate : Concatenate  NumInputs=4
  conjugate_quaternion : Subsystem
      mask help: conjugate a quaternion
      mask Help:
      | Name:
      | 
      |     conjugate_quaternion
      | 
      | Description:
      | 
      |     computes the conjugate quaternion
      | 
      | Inputs  [size] [data type] [unit]:
      | 
      |     quaternion q_2_1  [4] [double] [-]
      | 
      | Outputs  [size] [data type] [unit]:
      | 
      |     conjugated quaternion q_1_2  [4] [double] [-]
      mask Display: disp (' conj(q)')
  conjugate_quaternion1 : Subsystem
      mask help: conjugate a quaternion
      mask Help:
      | Name:
      | 
      |     conjugate_quaternion
      | 
      | Description:
      | 
      |     computes the conjugate quaternion
      | 
      | Inputs  [size] [data type] [unit]:
      | 
      |     quaternion q_2_1  [4] [double] [-]
      | 
      | Outputs  [size] [data type] [unit]:
      | 
      |     conjugated quaternion q_1_2  [4] [double] [-]
      mask Display: disp (' conj(q)')
  d_qIB : Outport  VectorParamsAs1DForOutWhenUnconnected=off
  wires:
  Q_3/1 -> Product4/1
  Add/1 -> Product6/1  "Q(w')"
  Demux1/1 -> Product2/2  "w1"
  Product5/1 -> Add/4
  Product6/1 -> Gain/1
  Q_4/1 -> Product5/1
  Demux1/2 -> Product3/2  "w2"
  Q_1/1 -> Product2/1
  Q_2/1 -> Product3/1
  Product3/1 -> Add/2
  Demux1/3 -> Product4/2  "w3"
  Demux1/4 -> Product5/2  "w4"
  Product4/1 -> Add/3
  Product2/1 -> Add/1
  Gain/1 -> conjugate_quaternion1/1(q)  "d_qBI"
  qIB/1 -> conjugate_quaternion/1(q)
  wBIB/1 -> Demux/1
  Demux/1 -> Vector Concatenate/1
  Demux/2 -> Vector Concatenate/2
  Demux/3 -> Vector Concatenate/3
  Constant/1 -> Vector Concatenate/4
  Vector Concatenate/1 -> Demux1/1
  conjugate_quaternion/1(q_conj) -> Product6/2  "qBI"
  conjugate_quaternion1/1(q_conj) -> d_qIB/1  "d_qIB"

== system lib_FDM/FDM/FDM_Sophisticated/rb_eom/eom_6dof/Rigid_Body_EOM_6_DOF/rb_eom_6dof/cross_product ==
  note: Inputs [size]:
      |
      | r1 [3x1]
      | r2 [3x1]
  note: Outputs [size]:
      |
      | r1 x r2  [3x1]
  r1 : Inport
  r2 : Inport  Port=2
  Demux2 : Demux  Outputs=[1;1;1]
  Demux3 : Demux  Outputs=[1;1;1]
  Product{2..7} (6 alike) : Product  SaturateOnIntegerOverflow=on  RndMeth=Zero  InputSameDT=on  OutDataTypeStr=Inherit: Same as first input
  Sum : Sum  Inputs=+-  SaturateOnIntegerOverflow=on  InputSameDT=on  OutDataTypeStr=Inherit: Same as first input
  Sum1 : Sum  Inputs=+-  SaturateOnIntegerOverflow=on  InputSameDT=on  OutDataTypeStr=Inherit: Same as first input
  Sum2 : Sum  Inputs=+-  SaturateOnIntegerOverflow=on  InputSameDT=on  OutDataTypeStr=Inherit: Same as first input
  Vector Concatenate : Concatenate  NumInputs=3  Mode=Multidimensional array
  r1_x_r2 : Outport  PortDimensions=[3,1]  VectorParamsAs1DForOutWhenUnconnected=off
  wires:
  Vector Concatenate/1 -> r1_x_r2/1
  r2/1 -> Demux3/1
  r1/1 -> Demux2/1
  Sum2/1 -> Vector Concatenate/3
  Sum1/1 -> Vector Concatenate/2
  Sum/1 -> Vector Concatenate/1
  Product7/1 -> Sum2/2
  Product6/1 -> Sum2/1
  Product5/1 -> Sum1/2
  Product4/1 -> Sum1/1
  Product3/1 -> Sum/2
  Product2/1 -> Sum/1
  Demux2/1 -> Product5/1, Product6/1
  Demux3/1 -> Product4/2, Product7/2
  Demux2/3 -> Product4/1, Product3/1
  Demux3/2 -> Product3/2, Product6/2
  Demux3/3 -> Product2/2, Product5/2
  Demux2/2 -> Product7/1, Product2/1

== system lib_FDM/FDM/FDM_Sophisticated/rb_eom/eom_6dof/Rigid_Body_EOM_6_DOF/rb_eom_6dof/r2_from_r1_trans_q21 ==
  note: Inputs [size]:
      |
      | vector r1 [3]
      | quaternion q21 [4]
  note: Outputs [size]:
      |
      | vector r2 [3]
  r1 : Inport
  q21 : Inport  Port=2
  Add : Sum  Inputs=++++
  Add1 : Sum  Inputs=++++
  Constant : Constant  Value=0
  Demux : Demux  Outputs=3
  Demux1 : Demux
  Demux2 : Demux
  Math Function : Math  Operator=transpose  SaturateOnIntegerOverflow=on
  Product{,1..7} (8 alike) : Product
  Product8 : Product  Inputs=3  Multiplication=Matrix(*)
  Q_1 : Constant  Value=[0 0 0 1; 0 0 1 0; 0 -1 0 0; -1 0 0 0]
  Q_2 : Constant  Value=[0 0 -1 0; 0 0 0 1; 1 0 0 0; 0 -1 0 0]
  Q_3 : Constant  Value=[0 1 0 0; -1 0 0 0; 0 0 0 1; 0 0 -1 0]
  Q_4 : Constant  Value=[1 0 0 0; 0 1 0 0; 0 0 1 0; 0 0 0 1]
  Q~_1 : Constant  Value=[0 0 0 1; 0 0 -1 0; 0 1 0 0; -1 0 0 0]
  Q~_2 : Constant  Value=[0 0 1 0; 0 0 0 1; -1 0 0 0; 0 -1 0 0]
  Q~_3 : Constant  Value=[0 -1 0 0; 1 0 0 0; 0 0 0 1; 0 0 -1 0]
  Q~_4 : Constant  Value=[1 0 0 0; 0 1 0 0; 0 0 1 0; 0 0 0 1]
  Selector : Selector  IndexMode=Zero-based  InputPortWidth=4  IndexOptions=Index vector (dialog)  Indices=[0 1 2]  OutputSizes=1
  Vector Concatenate : Concatenate  NumInputs=4
  r2 : Outport  VectorParamsAs1DForOutWhenUnconnected=off
  wires:
  r1/1 -> Demux/1
  Demux/1 -> Vector Concatenate/1  "rx"
  Demux/2 -> Vector Concatenate/2  "ry"
  Demux/3 -> Vector Concatenate/3  "rz"
  Demux1/1 -> Product/2  "q1"
  Demux1/2 -> Product1/2  "q2"
  Demux1/3 -> Product2/2  "q3"
  Demux1/4 -> Product3/2  "q4"
  Q_1/1 -> Product/1
  Q_2/1 -> Product1/1
  Q_3/1 -> Product2/1
  Q_4/1 -> Product3/1
  Product/1 -> Add/1
  Product1/1 -> Add/2
  Product2/1 -> Add/3
  Product3/1 -> Add/4
  Add/1 -> Product8/2  "Q(q)"
  Demux2/1 -> Product4/2  "q1"
  Demux2/4 -> Product7/2  "q4"
  Q~_2/1 -> Product5/1
  Product4/1 -> Add1/1
  Product7/1 -> Add1/4
  q21/1 -> Demux2/1, Demux1/1
  Add1/1 -> Math Function/1  "Q~(q)"
  Demux2/2 -> Product5/2  "q2"
  Product5/1 -> Add1/2
  Demux2/3 -> Product6/2  "q3"
  Product6/1 -> Add1/3
  Q~_4/1 -> Product7/1
  Q~_1/1 -> Product4/1
  Q~_3/1 -> Product6/1
  Math Function/1 -> Product8/1  "Q~T(q)"
  Constant/1 -> Vector Concatenate/4
  Vector Concatenate/1 -> Product8/3
  Product8/1 -> Selector/1
  Selector/1 -> r2/1

== system lib_FDM/FDM/FDM_Sophisticated/stream_flow/calc_stream_flow/Subsystem1/AoA_Sideslip_Alphatot_Phi/norm_of_vector ==
  note: Inputs [size]:
      |
      | vector  [3]
  note: Outputs [size]:
      |
      | norm of vector [1]
  vector : Inport
  Dot Product1 : DotProduct  InputSameDT=on  OutDataTypeStr=Inherit: Inherit via internal rule
  Math Function1 : Math  Operator=sqrt  SaturateOnIntegerOverflow=on
  norm_of_vector : Outport  VectorParamsAs1DForOutWhenUnconnected=off
  wires:
  Dot Product1/1 -> Math Function1/1
  Math Function1/1 -> norm_of_vector/1
  vector/1 -> Dot Product1/2, Dot Product1/1

== system lib_FDM/FDM/FDM_Sophisticated/tmp/weather/atm_dynamic/trafo_around_z_axis/1_rot_mat ==
  wi1 : Inport
  1. Rotation x-Achse : Subsystem
  1. Rotation y-Achse : Subsystem
  1. Rotation z-Achse : Subsystem
  Constant : Constant  Value=rot_1
  Multiport Switch : MultiPortSwitch
  T12 : Outport  VectorParamsAs1DForOutWhenUnconnected=off
  wires:
  Multiport Switch/1 -> T12/1  "T12"
  wi1/1 -> 1. Rotation y-Achse/1(alpha1), 1. Rotation z-Achse/1(alpha1), 1. Rotation x-Achse/1(alpha1)
  1. Rotation z-Achse/1(1Rot_Matrix_z) -> Multiport Switch/4
  1. Rotation y-Achse/1(1Rot_Matrix_y) -> Multiport Switch/3
  1. Rotation x-Achse/1(1Rot_Matrix_x) -> Multiport Switch/2
  Constant/1 -> Multiport Switch/1

== system lib_FDM/FDM/FDM_Sophisticated/weight_and_balance/moi/moi_coordinate_transformation/3_rot_mat/1. Rotation x-Achse ==
  alpha1 : Inport
  Constant : Constant
  Constant{1..2,7..8} (4 alike) : Constant  Value=0
  Gain : Gain  Gain=-1
  Matrix Concatenate : Concatenate  NumInputs=3  Mode=Multidimensional array  ConcatenateDimension=2
  Mux : Mux  Inputs=3
  Mux1 : Mux  Inputs=3
  Mux2 : Mux  Inputs=3
  Trigonometric Function : Trigonometry  Operator=cos
  Trigonometric Function1 : Trigonometry
  Trigonometric Function2 : Trigonometry
  Trigonometric Function3 : Trigonometry  Operator=cos
  1Rot_Matrix_x : Outport  VectorParamsAs1DForOutWhenUnconnected=off
  wires:
  Matrix Concatenate/1 -> 1Rot_Matrix_x/1
  Mux2/1 -> Matrix Concatenate/3
  Mux1/1 -> Matrix Concatenate/2
  Mux/1 -> Matrix Concatenate/1
  Trigonometric Function3/1 -> Mux2/3
  Trigonometric Function1/1 -> Mux2/2
  Constant7/1 -> Mux2/1
  Trigonometric Function2/1 -> Gain/1
  Trigonometric Function/1 -> Mux1/2
  Constant8/1 -> Mux1/1
  Constant2/1 -> Mux/3
  Constant1/1 -> Mux/2
  Constant/1 -> Mux/1
  alpha1/1 -> Trigonometric Function3/1, Trigonometric Function1/1, Trigonometric Function/1, Trigonometric Function2/1
  Gain/1 -> Mux1/3

== system lib_FDM/FDM/FDM_Sophisticated/weight_and_balance/moi/moi_coordinate_transformation/3_rot_mat/1. Rotation y-Achse ==
  alpha1 : Inport
  Constant{,2,7..8} (4 alike) : Constant  Value=0
  Constant1 : Constant
  Gain1 : Gain  Gain=-1
  Matrix Concatenate : Concatenate  NumInputs=3  Mode=Multidimensional array  ConcatenateDimension=2
  Mux : Mux  Inputs=3
  Mux1 : Mux  Inputs=3
  Mux2 : Mux  Inputs=3
  Trigonometric Function : Trigonometry  Operator=cos
  Trigonometric Function1 : Trigonometry
  Trigonometric Function2 : Trigonometry
  Trigonometric Function3 : Trigonometry  Operator=cos
  1Rot_Matrix_y : Outport  VectorParamsAs1DForOutWhenUnconnected=off
  wires:
  Matrix Concatenate/1 -> 1Rot_Matrix_y/1
  Constant7/1 -> Mux2/2
  Trigonometric Function2/1 -> Mux/3
  Trigonometric Function/1 -> Mux/1
  Constant8/1 -> Mux/2
  alpha1/1 -> Trigonometric Function/1, Trigonometric Function2/1, Trigonometric Function3/1, Trigonometric Function1/1
  Constant/1 -> Mux1/1
  Constant1/1 -> Mux1/2
  Constant2/1 -> Mux1/3
  Trigonometric Function1/1 -> Gain1/1
  Trigonometric Function3/1 -> Mux2/3
  Mux/1 -> Matrix Concatenate/1
  Mux1/1 -> Matrix Concatenate/2
  Mux2/1 -> Matrix Concatenate/3
  Gain1/1 -> Mux2/1
